simulink model "fir"  (R2018a)
settings: Solver=VariableStepAuto  StartTime=0.0  StopTime=0.0005  RelTol=1e-3
libraries: xbsIndex_r4 x4
settings Model: Creator=57315  LastModifiedBy=57315

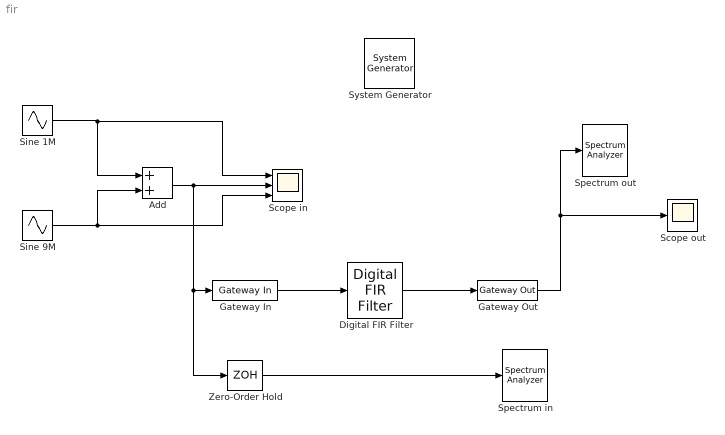
== system fir ==
  " System Generator" : xbsIndex_r4/ System Generator  Tag=genX  xilinxfamily=zynq  part=xc7z010  speed=-1  package=clg400  synthesis_tool=Vivado  clock_wrapper=Clock Enables  directory=C:/a_max/max_xilinx/max/System_Generator/FIR  proj_type=Vivado  Synth_file=Vivado Synthesis Defaults  Impl_file=Vivado Implementation Defaults  testbench=on  simulink_period=1/20e6  sysclk_period=50  dcm_input_clock_period=10  incr_netlist=off  trim_vbits=Everywhere in SubSystem  dbl_ovrd=According to Block Masks  core_generation=According to Block Masks  run_coregen=off  deprecated_control=off  eval_field=0  block_type=sysgen
  Add : Sum
  Digital FIR Filter : xbsIndex_r4/Digital FIR Filter  coeff_source=on  coefficientvector=fir1(15,0.5)  coeff_calulate=on  coefficient_width=19  coefficient_fractional_bits=19  interpolation_filter_rate=1  decimation_filter_rate=1  fda_coefficientvector=[0.00190671341889057 -0.0110752394328746 -0.04115159144813 0.0351305675326196 0.288782784611287 0.450932479760355 0.288782784611287 0.0351305675326196 -0.04115159144813 -0.0110752394328746 0.00190671341889057]  simulation_type=fast_sim  simulation_model=sysgen:fir_macro  block_type=fir_macro
  Gateway In : xbsIndex_r4/Gateway In  gui_display_data_type=Fixed-point  arith_type="Signed  (2's comp)"  n_bits=32  bin_pt=30  preci_type=Single  exp_width=8  frac_width=24  rows=1  columns=1  quantization="Round  (unbiased: +/- Inf)"  overflow=Saturate  period=1/20e6  UseAsADC=off  ADCChannel='1'  interface=None  automatic_assignment=on  address_offset=hex2dec('00')  intf_name=''  intf_description=''  default_value=0  timing_constraint=None  locs_specified=off  LOCs={}  io_standard={}  inherit_from_input=off  hdl_port=on  dbl_ovrd=off  block_type=gatewayin
  Gateway Out : xbsIndex_r4/Gateway Out  inherit_from_input=off  hdl_port=on  rows=1  columns=1  UseAsDAC=off  DACChannel='1'  interface=None  automatic_assignment=on  address_offset=hex2dec('00')  intf_name=''  intf_description=''  timing_constraint=None  locs_specified=off  LOCs={}  io_standard={}  block_type=gatewayout
  Scope in : Scope  NumInputPorts=3
  Scope out : Scope  NumInputPorts=3
  Sine 1M : Sin  Frequency=2*pi*1e6  SampleTime=0
  Sine 9M : Sin  Frequency=2*pi*9e6  SampleTime=0
  "Spectrum in " : SpectrumAnalyzer
  Spectrum out : SpectrumAnalyzer
  Zero-Order Hold : ZeroOrderHold  SampleTime=1/20e6
  wires:
  Sine 1M/1 -> Scope in/1, Add/1
  Sine 9M/1 -> Scope in/3, Add/2
  Gateway In/1 -> Digital FIR Filter/1
  Add/1 -> Zero-Order Hold/1, Gateway In/1, Scope in/2
  Digital FIR Filter/1 -> Gateway Out/1
  Zero-Order Hold/1 -> "Spectrum in "/1
  Gateway Out/1 -> Scope out/2, Spectrum out/1
